simulink model "DynamiquePlaque"  (R2018b)
settings: Solver=VariableStepAuto  StartTime=0.0  StopTime=10.0  RelTol=1e-3
values from neighbouring files (symbols this model uses):
  g = 9.81    [Modele.m]
  XA = r_abc    (= 0.0952)    [Modele.m]
  XB = -r_abc*sind(30)    [Modele.m]
  XC = -r_abc*sind(30)    [Modele.m]
  YB = r_abc*cosd(30)    [Modele.m]
  YC = -r_abc*cosd(30)    [Modele.m]
undefined symbols (not defined in the file or in its folder): Jx, Jy, mSg, mtot
libraries: dspsrcs4 x2
settings Model: Creator=Vincent  LastModifiedBy=Vincent

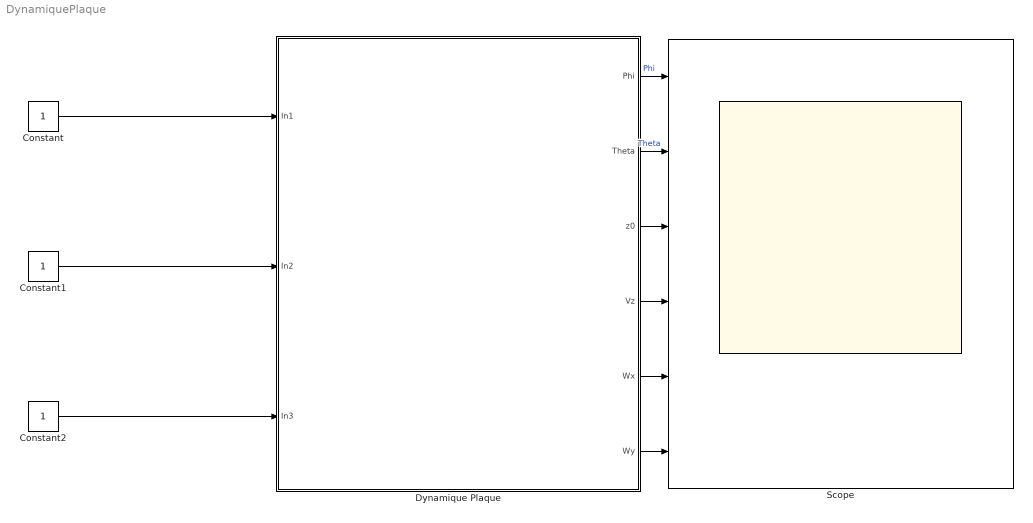
== system DynamiquePlaque ==
  Constant : Constant
  Constant1 : Constant
  Constant2 : Constant
  Dynamique Plaque : Subsystem
  Scope : Scope  NumInputPorts=6
  wires:
  Constant1/1 -> Dynamique Plaque/2(In2)
  Constant/1 -> Dynamique Plaque/1(In1)
  Constant2/1 -> Dynamique Plaque/3(In3)
  Dynamique Plaque/1(Phi) -> Scope/1  "Phi"
  Dynamique Plaque/2(Theta) -> Scope/2  "Theta"
  Dynamique Plaque/3(z0) -> Scope/3
  Dynamique Plaque/4(Vz) -> Scope/4
  Dynamique Plaque/5(Wx) -> Scope/5
  Dynamique Plaque/6(Wy) -> Scope/6

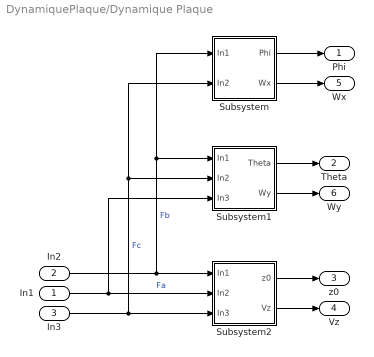
== system DynamiquePlaque/Dynamique Plaque ==
  In1 : Inport
  In2 : Inport  Port=2
  In3 : Inport  Port=3
  Subsystem : Subsystem
  Subsystem1 : Subsystem
  Subsystem2 : Subsystem
  Phi : Outport
  Theta : Outport  Port=2
  z0 : Outport  Port=3
  Vz : Outport  Port=4
  Wx : Outport  Port=5
  Wy : Outport  Port=6
  wires:
  In1/1 -> Subsystem1/3(In3), Subsystem2/2(In2)  "Fa"
  In3/1 -> Subsystem/2(In2), Subsystem1/2(In2), Subsystem2/3(In3)  "Fc"
  Subsystem1/1(Theta) -> Theta/1
  In2/1 -> Subsystem1/1(In1), Subsystem/1(In1), Subsystem2/1(In1)  "Fb"
  Subsystem/1(Phi) -> Phi/1
  Subsystem2/1(z0) -> z0/1
  Subsystem2/2(Vz) -> Vz/1
  Subsystem/2(Wx) -> Wx/1
  Subsystem1/2(Wy) -> Wy/1

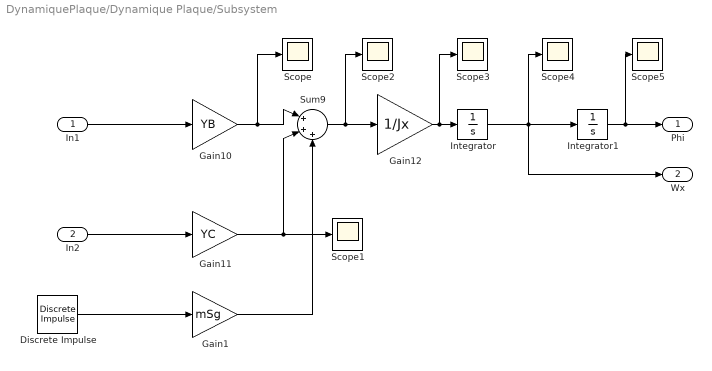
== system DynamiquePlaque/Dynamique Plaque/Subsystem ==
  In1 : Inport
  In2 : Inport  Port=2
  Discrete Impulse : dspsrcs4/Discrete  Impulse  Delay=0  SampleTime=1  FrameSample=1  OutputFrames=off  dataType=double  isSigned=on  wordLen=16  udDataType=sfix(16)  fracBitsMode=Best precision  numFracBits=15  OutDataTypeStr=double  LastOutDataTypeStr=double
  Gain1 : Gain  Gain=mSg
  Gain10 : Gain  Gain=YB
  Gain11 : Gain  Gain=YC
  Gain12 : Gain  Gain=1/Jx
  Integrator : Integrator
  Integrator1 : Integrator
  Scope{,1..5} (6 alike) : Scope
  Sum9 : Sum  Inputs=|+++
  Phi : Outport
  Wx : Outport  Port=2
  wires:
  Integrator1/1 -> Scope5/1, Phi/1
  In2/1 -> Gain11/1
  Integrator/1 -> Scope4/1, Wx/1, Integrator1/1
  Gain10/1 -> Scope/1, Sum9/1
  Sum9/1 -> Scope2/1, Gain12/1
  Gain11/1 -> Scope1/1, Sum9/2
  In1/1 -> Gain10/1
  Gain12/1 -> Scope3/1, Integrator/1
  Discrete Impulse/1 -> Gain1/1
  Gain1/1 -> Sum9/3

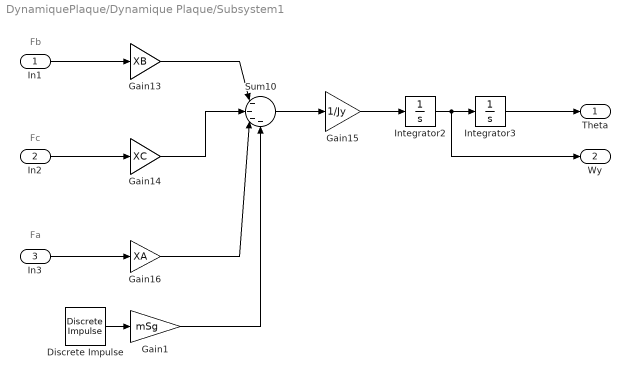
== system DynamiquePlaque/Dynamique Plaque/Subsystem1 ==
  note: Fa
  note: Fc
  note: Fb
  In1 : Inport
  In2 : Inport  Port=2
  In3 : Inport  Port=3
  Discrete Impulse : dspsrcs4/Discrete  Impulse  Delay=0  SampleTime=1  FrameSample=1  OutputFrames=off  dataType=double  isSigned=on  wordLen=16  udDataType=sfix(16)  fracBitsMode=Best precision  numFracBits=15  OutDataTypeStr=double  LastOutDataTypeStr=double
  Gain1 : Gain  Gain=mSg
  Gain13 : Gain  Gain=XB
  Gain14 : Gain  Gain=XC
  Gain15 : Gain  Gain=1/Jy
  Gain16 : Gain  Gain=XA
  Integrator2 : Integrator
  Integrator3 : Integrator
  Sum10 : Sum  Inputs=|----
  Theta : Outport
  Wy : Outport  Port=2
  wires:
  In3/1 -> Gain16/1
  Gain14/1 -> Sum10/2
  Gain15/1 -> Integrator2/1
  Sum10/1 -> Gain15/1
  Integrator2/1 -> Wy/1, Integrator3/1
  In1/1 -> Gain13/1
  Gain13/1 -> Sum10/1
  Integrator3/1 -> Theta/1
  Gain16/1 -> Sum10/3
  In2/1 -> Gain14/1
  Gain1/1 -> Sum10/4
  Discrete Impulse/1 -> Gain1/1

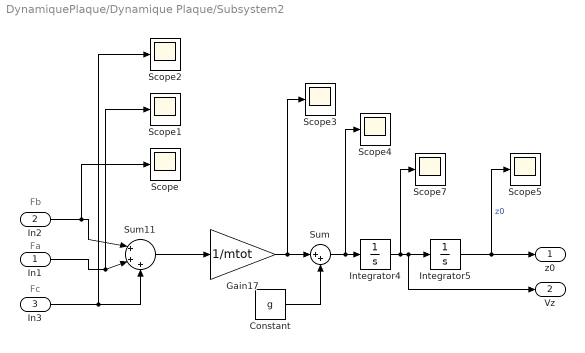
== system DynamiquePlaque/Dynamique Plaque/Subsystem2 ==
  note: Fc
  note: Fa
  note: Fb
  In1 : Inport
  In2 : Inport  Port=2
  In3 : Inport  Port=3
  Constant : Constant  Value=g
  Gain17 : Gain  Gain=1/mtot
  Integrator4 : Integrator
  Integrator5 : Integrator
  Scope{,1..5,7} (7 alike) : Scope
  Sum : Sum  Inputs=|++
  Sum11 : Sum  Inputs=|+++
  z0 : Outport
  Vz : Outport  Port=2
  wires:
  Integrator5/1 -> Scope5/1, z0/1  "z0"
  In3/1 -> Scope2/1, Sum11/3
  Sum11/1 -> Gain17/1
  In1/1 -> Scope1/1, Sum11/2
  Integrator4/1 -> Scope7/1, Vz/1, Integrator5/1
  Gain17/1 -> Scope3/1, Sum/1
  In2/1 -> Scope/1, Sum11/1
  Sum/1 -> Scope4/1, Integrator4/1
  Constant/1 -> Sum/2
